simulink model "TireModelTestHarness"  (R2025b)
settings: Solver=VariableStepAuto  StartTime=0.0  StopTime=20  RelTol=1e-3
libraries: fl_lib x13, nesl_utility x2, sdl_lib x1
settings Model: Creator=asakhare  LastModifiedBy=varora
settings SimscapeCC: SimscapeLogType=all

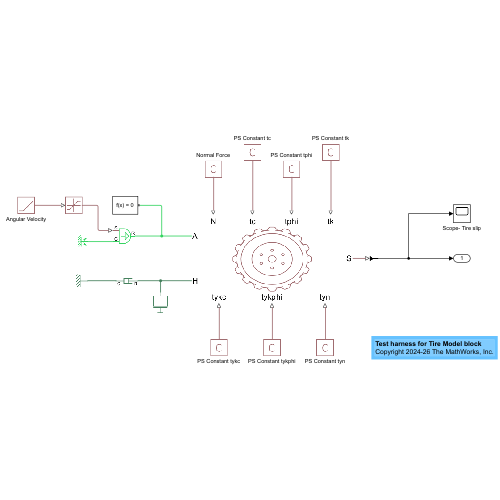
[thumbnail: Simulink's stored preview of the top-level diagram]
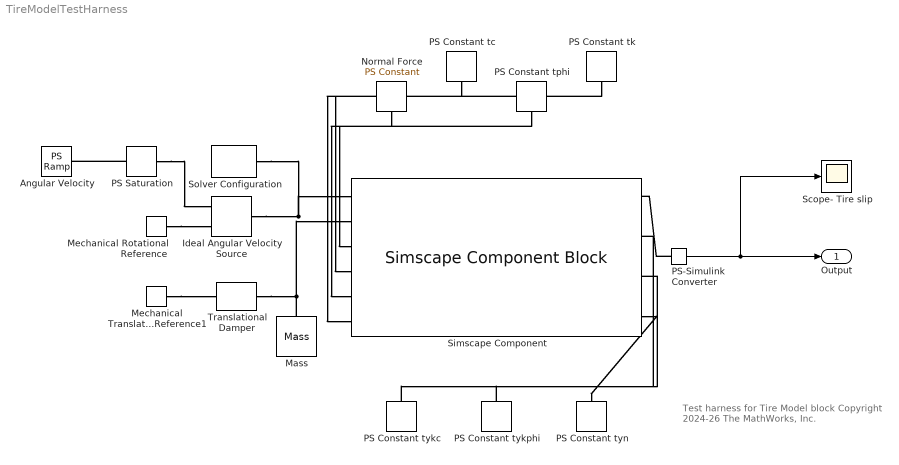
== system TireModelTestHarness ==
  note: Test harness for Tire Model block
      | Copyright 2024-26 The MathWorks, Inc.
  Angular Velocity : fl_lib/Physical Signals/Sources/PS Ramp  slope=6 rad/s^2  start_time=0.5 s  initial_output=0 rad/s  ZeroCross=true
  Ideal Angular Velocity Source : fl_lib/Mechanical/Mechanical Sources/Ideal Angular Velocity Source
  Mass : fl_lib/Mechanical/Translational Elements/Mass  mass=10 kg  num_ports=foundation.enum.numPorts2.one  v_specify=off  v_priority=High  v=.5 m/s  v_nominal_specify=off  v_nominal_value=1  v_nominal_unit=m/s  f_specify=off  f_priority=None  f=0 N  f_nominal_specify=off  f_nominal_value=1  f_nominal_unit=N
  Mechanical Rotational Reference : fl_lib/Mechanical/Rotational Elements/Mechanical Rotational Reference
  Mechanical Translational Reference1 : fl_lib/Mechanical/Translational Elements/Mechanical Translational Reference
  Normal Force : fl_lib/Physical Signals/Sources/PS Constant  constant=1000 N
  PS Constant tc : fl_lib/Physical Signals/Sources/PS Constant  constant=1000 N/m^2
  PS Constant tk : fl_lib/Physical Signals/Sources/PS Constant  constant=0.1 m
  PS Constant tphi : fl_lib/Physical Signals/Sources/PS Constant  constant=60 deg
  PS Constant tykc : fl_lib/Physical Signals/Sources/PS Constant  constant=48
  PS Constant tykphi : fl_lib/Physical Signals/Sources/PS Constant  constant=6067
  PS Constant tyn : fl_lib/Physical Signals/Sources/PS Constant  constant=0.78
  PS Saturation : fl_lib/Physical Signals/Nonlinear Operators/PS Saturation  upper_limit=30 rad/s  lower_limit=-30 rad/s  ZeroCross=true
  PS-Simulink Converter : nesl_utility/PS-Simulink Converter  PhysicalDomain=network_engine_domain  SubClassName=ps_output  LeftPortType=input  RightPortType=output  PseudoPeriodic=off  Frequencies=[]  VectorFormat=inherit  Unit=inherit  AffineConversion=off
  Scope- Tire slip : Scope
  Simscape Component : SimscapeComponentBlock  SourceFile=tire_soil  ComponentPath=tire_soil  ComponentVariants="[\"tire_soil\"]"  ComponentVariantNames="[\"tire_soil\"]"  ClassName=tire_soil  SchemaVersion=1  load_TLU=[2.225, 4.45, 6.6725, 8.9, 11.125, 13.35] kN  p_inflation_TLU=[69, 138, 207, 276, 345] kPa  deflection_TLU=[1.896, 1.239, 1.021, .894, .776; 3.623, 2.423, 1.963, 1.64, 1.435; 5.119, 3.477, 2.77, 2.311, 2.008; 6.447, 4.413, 3.528, 2.939, 2.533; 7.917, 5.306, 4.191, 2.494, 3.03; 9.169, 6.098, 4.851, 4.059, 3.494] cm  area_TLU=[179.93, 145.82, 127.81, 102.68, 100.92; 517.26, 262.89, 211.79, 182.92, 165.86; 726.09, 424.44, 304.42, 241.47, 233.76; 947.36, 604.21, 414.85, 343.35, 297.14; 1085.95, 749.58, 556.91, 443.03, 372.77; 1214.12, 865.65, 649.45, 525.61, 445.5] cm^2  inflation_pressure=100 kPa  k_e=7  r_e=0.5 m  bti=0.327 m  hti=0.245 m  model_compliance=sdl.enum.compliance.on  stiffness=1e6 N/m  damping=1000 N*s/m  model_inertia=sdl.enum.model_inertia.on  inertia=1 kg*m^2  initial_velocity=0 rad/s  vxlow=1 m/s  v_tr_thr=0.001 m/s  kpumin=-1  kpumax=1  p_thr=0.01 bar  b_thr=1 mm  r_e_t=0.5 m  rolling_radius_model=sdl.enum.RollingRadiusParameterization.Constant  fz0=4000 N  r_0=0.5 m  breff=8.39  dreff=0.26  freff=0.074  q_re0=0.99  q_v1=0.008  longvl=17 m/s  cz=5e5 N/m
      settings: CopyFcn=simscape.sscblock.internal.componentBlockCallback(gcbh,'COPY')  PreCopyFcn=simscape.sscblock.internal.componentBlockCallback(gcbh,'PRECOPY')  PreDeleteFcn=simscape.sscblock.internal.componentBlockCallback(gcbh,'PREDELETE')  InternalSimscapePortConfiguration="{\"Bottom\":[{\"id\":\"tykc\",\"label\":\"tykc\",\"type\":\"input\"},{\"id\":\"tykphi\",\"label\":\"tykphi\",\"type\":\"input\"},{\"id\":\"tyn\",\"label\":\"tyn\",\"type\":\"input\"}],\"Left\":[{\"id\":\"A\",\"label\":\"A\",\"type\":\"foundation.mechanical.rotational.rotational\"},{\"id\":\"H\",\"label\":\"H\",\"type\":\"foundation.mechanical.translational.translational\"}],\"Right\":[{\"id\":\"S\",\"label\":\"S\",\"type\":\"output\"}],\"Top\":[{\"id\":\"N\",\"label\":\"N\",\"type\":\"input\"},{\"id\":\"tc\",\"label\":\"tc\",\"type\":\"input\"},{\"id\":\"tphi\",\"label\":\"tphi\",\"type\":\"input\"},{\"id\":\"tk\",\"label\":\"tk\",\"type\":\"input\"}]}"
      mask Type: Tire (Tire-Soil)
  Solver Configuration : nesl_utility/Solver Configuration  PhysicalDomain=network_engine_domain  SubClassName=solver  LeftPortType=input  RightPortType=generic  Tones=[]  Harmonics=[]  SimulateNoise=off  Profile=off  UseLocalSampling=off  EnableSwitchedLinearOptims=on  FrequencyDomain=off  UseCCode=off  RelTol=0.001  AbsTol=0.001  MinStep=1e-09  ToWorkspace=off  RevertToSquareIcSolve=off  NumHomotopyIterations=100  PhasorMode=off  PhasorModeNumHarmonics=1  ConsistencySolver=NEWTON_XTOL_AFTER_FTOL  IndexReductionMethod=DerivativeReplacement  DoDC=off  ResidualTolerance=1e-09  ConsistencyTolSource=GLOBAL  ConsistencyAbsTol=0.001  ConsistencyRelTol=0.001  ConsistencyTolFactor=0.001  UseLocalSolver=off  LocalSolverChoice=NE_BACKWARD_EULER_ADVANCER  ResolveIndetEquations=on  FunctionEvalNumThread=1  LocalSolverSampleTime=0.001  DoFixedCost=off  MaxNonlinIter=3  MaxModeIter=2  ComputeImpulses=off  ImpulseIterations=2  LinearAlgebra=auto  LinearAlgebraNumThread=0  EquationFormulation=NE_TIME_EF  DelaysMemoryBudget=1024  AutomaticFiltering=on  FilteringTimeConstant=0.001  PartitionStorageMethod=AS_NEEDED  PartitionMemoryBudget=1024  PartitionMethod=ROBUST  MultibodyUseLocalSolver=off  MultibodyLocalSolverChoice=ODE1  MultibodyLocalSolverSampleTime=0.001
  Translational Damper : sdl_lib/Couplings & Drives/Springs & Dampers/Translational Damper  D=1e-3 N*s/m  thermal_port=simscape.enum.thermaleffects.omit  thermal_mass=50 kJ/K  temperature_specify=off  temperature_priority=High  temperature=300 K  temperature_nominal_specify=off  temperature_nominal_value=1  temperature_nominal_unit=K
  Output : Outport
  wires:
  PS-Simulink Converter/1 -> Scope- Tire slip/1, Output/1
  connections:
  Normal Force/RConn1 -- Simscape Component/LConn3
  PS Constant tc/RConn1 -- Simscape Component/LConn4
  PS Constant tphi/RConn1 -- Simscape Component/LConn5
  PS Constant tk/RConn1 -- Simscape Component/LConn6
  PS Constant tykc/RConn1 -- Simscape Component/RConn2
  PS Constant tykphi/RConn1 -- Simscape Component/RConn3
  Simscape Component/RConn4 -- PS Constant tyn/RConn1
  Mass/LConn1 -- Simscape Component/LConn2 -- Translational Damper/LConn1
  Mechanical Translational Reference1/LConn1 -- Translational Damper/RConn1
  Ideal Angular Velocity Source/LConn1 -- Solver Configuration/RConn1 -- Simscape Component/LConn1
  Mechanical Rotational Reference/LConn1 -- Ideal Angular Velocity Source/RConn2
  PS Saturation/LConn1 -- Angular Velocity/RConn1
  PS Saturation/RConn1 -- Ideal Angular Velocity Source/RConn1
  PS-Simulink Converter/LConn1 -- Simscape Component/RConn1
